simulink library "GenTil_Lib"  (R2023a)
settings: Solver=VariableStepAuto  StartTime=0.0  StopTime=10.0  RelTol=1e-3
values from neighbouring files (symbols this model uses):
  D = [0	0	0	0	0	0	0	0	0	0	0 ... (first row only)    [GenTil.m]
undefined symbols (not defined in the file or in its folder): aircraft, p, phi, psi, q, r, theta, v, w, x, y, z
libraries: simulink_extras x35, simulink x5, matrix_library x4, aerolibatmos2 x1
(part 1 of 2)
settings Model: Creator=igmso  LastModifiedBy=igmso

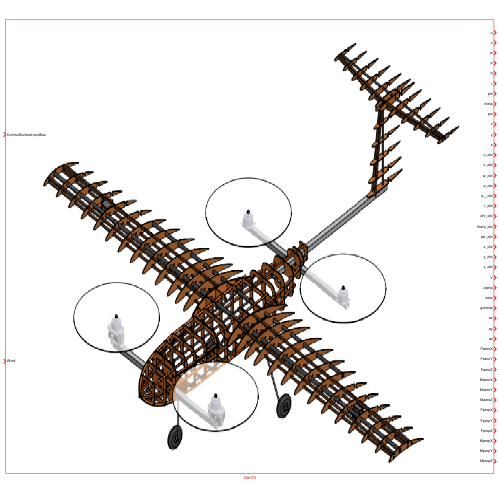
[thumbnail: Simulink's stored preview of the top-level diagram]
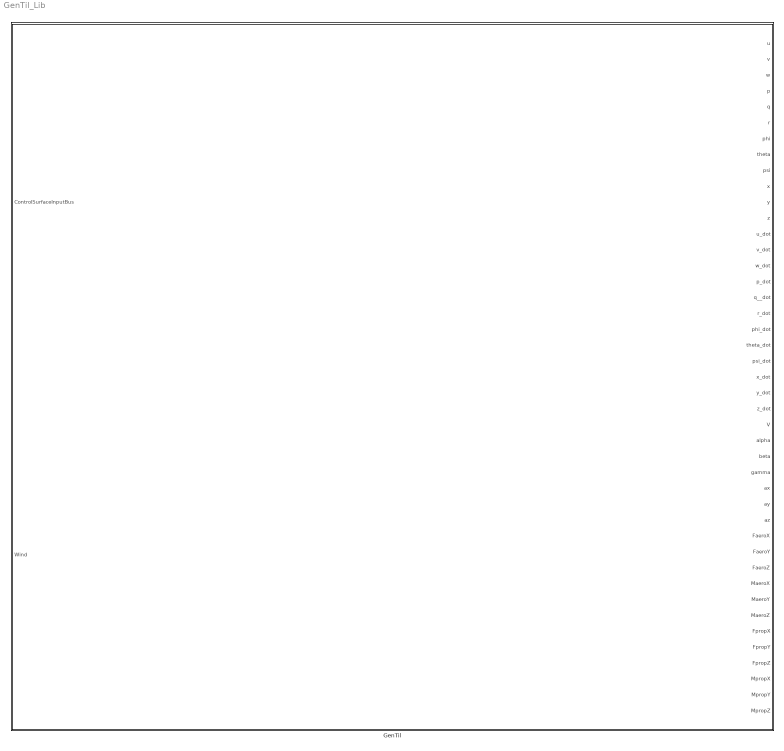
== system GenTil_Lib ==
  GenTil : Subsystem
      mask Display: image('Tilt.png'); % Use "Edit Image" on toolstrip to change.

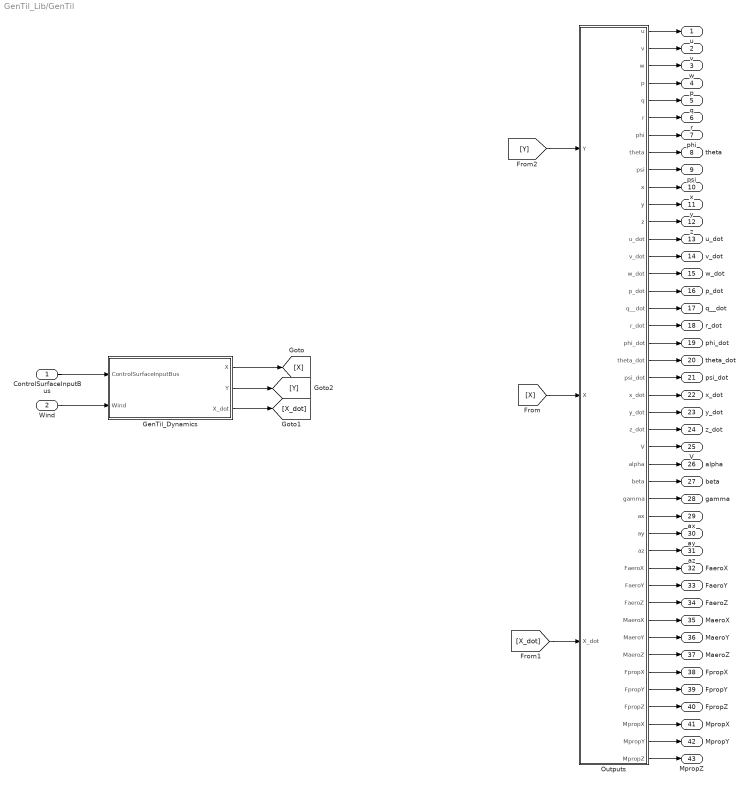
== system GenTil_Lib/GenTil ==
  ControlSurfaceInputBus : Inport  OutDataTypeStr=Bus: Actuators
  Wind : Inport  Port=2
  GenTil_Dynamics : Subsystem
  Outputs : Subsystem
  u : Outport
  v : Outport  Port=2
  w : Outport  Port=3
  p : Outport  Port=4
  q : Outport  Port=5
  r : Outport  Port=6
  phi : Outport  Port=7
  theta : Outport  Port=8
  psi : Outport  Port=9
  x : Outport  Port=10
  y : Outport  Port=11
  z : Outport  Port=12
  u_dot : Outport  Port=13
  v_dot : Outport  Port=14
  w_dot : Outport  Port=15
  p_dot : Outport  Port=16
  q__dot : Outport  Port=17
  r_dot : Outport  Port=18
  phi_dot : Outport  Port=19
  theta_dot : Outport  Port=20
  psi_dot : Outport  Port=21
  x_dot : Outport  Port=22
  y_dot : Outport  Port=23
  z_dot : Outport  Port=24
  V : Outport  Port=25
  alpha : Outport  Port=26
  beta : Outport  Port=27
  gamma : Outport  Port=28
  ax : Outport  Port=29
  ay : Outport  Port=30
  az : Outport  Port=31
  FaeroX : Outport  Port=32
  FaeroY : Outport  Port=33
  FaeroZ : Outport  Port=34
  MaeroX : Outport  Port=35
  MaeroY : Outport  Port=36
  MaeroZ : Outport  Port=37
  FpropX : Outport  Port=38
  FpropY : Outport  Port=39
  FpropZ : Outport  Port=40
  MpropX : Outport  Port=41
  MpropY : Outport  Port=42
  MpropZ : Outport  Port=43
  wires:
  Outputs/40(FpropZ) -> FpropZ/1
  Outputs/12(z) -> z/1
  Outputs/8(theta) -> theta/1
  GenTil_Dynamics/1(X) -> [X]
  Outputs/1(u) -> u/1
  Outputs/19(phi_dot) -> phi_dot/1
  Outputs/20(theta_dot) -> theta_dot/1
  Outputs/3(w) -> w/1
  Outputs/27(beta) -> beta/1
  Outputs/39(FpropY) -> FpropY/1
  GenTil_Dynamics/2(Y) -> [Y]
  Outputs/6(r) -> r/1
  Outputs/31(az) -> az/1
  Outputs/33(FaeroY) -> FaeroY/1
  Outputs/23(y_dot) -> y_dot/1
  [X_dot] -> Outputs/3(X_dot)
  Outputs/2(v) -> v/1
  Outputs/9(psi) -> psi/1
  Outputs/30(ay) -> ay/1
  Outputs/41(MpropX) -> MpropX/1
  Outputs/11(y) -> y/1
  Outputs/18(r_dot) -> r_dot/1
  Outputs/34(FaeroZ) -> FaeroZ/1
  Outputs/16(p_dot) -> p_dot/1
  Outputs/24(z_dot) -> z_dot/1
  [Y] -> Outputs/1(Y)
  Outputs/37(MaeroZ) -> MaeroZ/1
  Outputs/43(MpropZ) -> MpropZ/1
  Outputs/35(MaeroX) -> MaeroX/1
  Outputs/13(u_dot) -> u_dot/1
  Outputs/28(gamma) -> gamma/1
  Outputs/26(alpha) -> alpha/1
  Outputs/5(q) -> q/1
  Outputs/42(MpropY) -> MpropY/1
  Outputs/29(ax) -> ax/1
  Outputs/7(phi) -> phi/1
  GenTil_Dynamics/3(X_dot) -> [X_dot]
  [X] -> Outputs/2(X)
  Outputs/22(x_dot) -> x_dot/1
  Outputs/10(x) -> x/1
  Outputs/36(MaeroY) -> MaeroY/1
  Outputs/25(V) -> V/1
  Outputs/4(p) -> p/1
  Outputs/15(w_dot) -> w_dot/1
  Outputs/32(FaeroX) -> FaeroX/1
  ControlSurfaceInputBus/1 -> GenTil_Dynamics/1(ControlSurfaceInputBus)
  Outputs/38(FpropX) -> FpropX/1
  Wind/1 -> GenTil_Dynamics/2(Wind)
  Outputs/21(psi_dot) -> psi_dot/1
  Outputs/17(q__dot) -> q__dot/1
  Outputs/14(v_dot) -> v_dot/1

== system GenTil_Lib/GenTil/GenTil_Dynamics ==
  ControlSurfaceInputBus : Inport  OutDataTypeStr=Bus: Actuators
  Wind : Inport  Port=2
  Add1 : Sum  Inputs=+-
  Bus Creator : BusCreator  Inputs=2
  Bus Creator2 : BusCreator  Inputs=6
  Bus Creator5 : BusCreator  Inputs=19  OutDataTypeStr=Bus: Outs
      settings: InheritFromInputs=off
  Bus Selector : BusSelector  OutputSignals=theta
  Constant : Constant  Value=aircraft.m  OutDataTypeStr=double  SampleTime=-1
  Constant1 : Constant  Value=aircraft.J_O_b  VectorParams1D=off  OutDataTypeStr=double  SampleTime=-1
  Demux{1..2,4..6} (5 alike) : Demux  Outputs=3
  Demux3 : Demux  Outputs=6
  Equations_of_Motion_6DoF : Subsystem
  GenTilAeroProp : Subsystem
  Subsystem : Subsystem
  X : Outport  OutDataTypeStr=Bus: States
  Y : Outport  Port=2  OutDataTypeStr=Bus: Outs
  X_dot : Outport  Port=3
  wires:
  Bus Selector/1 -> [theta]  "<theta>"
  GenTilAeroProp/2(Moments) -> Demux1/1
  Demux6/3 -> Bus Creator2/3  "Zaero"
  Demux6/2 -> Bus Creator2/2  "Yaero"
  Demux1/1 -> Bus Creator2/4  "Laero"
  Constant/1 -> Bus Creator/1  "Mass_kg"
  Demux1/3 -> Bus Creator2/6  "Naero"
  Bus Creator2/1 -> Equations_of_Motion_6DoF/2(FromAero)  "FromAero"
  GenTilAeroProp/3(alpha) -> [alpha]  "alpha"
  GenTilAeroProp/5(V) -> [V]  "V"
  Constant1/1 -> Bus Creator/2  "InertiaTensor"
  ControlSurfaceInputBus/1 -> GenTilAeroProp/2(ControlSurfaceInputBus)  "Actuators"
  Bus Creator/1 -> Equations_of_Motion_6DoF/3(FromGeometry)  "FromGeometry"
  Demux6/1 -> Bus Creator2/1  "Xaero"
  Equations_of_Motion_6DoF/1(X) -> [X], Bus Selector/1  "X"
  GenTilAeroProp/4(beta) -> [beta]  "beta_"
  Wind/1 -> GenTilAeroProp/3(Wind)
  Subsystem/1(FromLG) -> Equations_of_Motion_6DoF/1(FromLG)
  GenTilAeroProp/6(n_C_b) -> [n_C_b]
  Demux5/3 -> Bus Creator5/18  "MpropZ"
  Demux2/1 -> Bus Creator5/4  "ax"
  Demux3/2 -> Bus Creator5/8  "FaeroY"
  Demux3/1 -> Bus Creator5/7  "FaeroX"
  [n_C_b] -> Demux2/1
  Add1/1 -> Bus Creator5/19  "gamma"
  Demux5/2 -> Bus Creator5/17  "MpropY"
  [alpha] -> Bus Creator5/2  "alpha"
  [V] -> Bus Creator5/1  "V"
  [FandM] -> Demux3/1
  Demux3/4 -> Bus Creator5/10  "MaeroX"
  Demux2/3 -> Bus Creator5/6  "az"
  [Fprop] -> Demux4/1
  Demux2/2 -> Bus Creator5/5  "ay"
  Demux5/1 -> Bus Creator5/16  "MpropX"
  Demux4/3 -> Bus Creator5/15  "FpropZ"
  [alpha] -> Add1/2  "alpha"
  [Mprop] -> Demux5/1
  Demux3/6 -> Bus Creator5/12  "MaeroZ"
  Bus Creator5/1 -> Y/1  "Outs"
  [beta] -> Bus Creator5/3  "beta"
  [theta] -> Add1/1
  Demux4/2 -> Bus Creator5/14  "FpropY"
  Demux4/1 -> Bus Creator5/13  "FpropX"
  Demux3/3 -> Bus Creator5/9  "FaeroZ"
  Demux3/5 -> Bus Creator5/11  "MaeroY"
  Equations_of_Motion_6DoF/2(X_dot) -> [Xdot]
  GenTilAeroProp/1(Forces) -> Demux6/1
  GenTilAeroProp/8(Fprop) -> [Fprop]
  GenTilAeroProp/7(Mprop) -> [Mprop]
  GenTilAeroProp/9(AeroCoeficients) -> [FandM]
  Demux1/2 -> Bus Creator2/5  "Maero"
  [X] -> Subsystem/1(X)
  [X] -> GenTilAeroProp/1(X)
  [X] -> X/1
  [Xdot] -> X_dot/1

== system GenTil_Lib/GenTil/Outputs ==
  Y : Inport  OutDataTypeStr=Bus: Outs
  X : Inport  Port=2  OutDataTypeStr=Bus: States
  X_dot : Inport  Port=3
  Bus Selector : BusSelector  OutputSignals=u,v,w,p,q,r,phi,theta,psi,x,y,z
  Bus Selector1 : BusSelector  OutputSignals=V,alpha,beta,gamma,ax,ay,az,FaeroX,FaeroY,FaeroZ,MaeroX,MaeroY,MaeroZ,FpropX,FpropY,FpropZ,MpropX,MpropY,MpropZ
  Demux1 : Demux  Outputs=12
  u : Outport
  v : Outport  Port=2
  w : Outport  Port=3
  p : Outport  Port=4
  q : Outport  Port=5
  r : Outport  Port=6
  phi : Outport  Port=7
  theta : Outport  Port=8
  psi : Outport  Port=9
  x : Outport  Port=10
  y : Outport  Port=11
  z : Outport  Port=12
  u_dot : Outport  Port=13
  v_dot : Outport  Port=14
  w_dot : Outport  Port=15
  p_dot : Outport  Port=16
  q__dot : Outport  Port=17
  r_dot : Outport  Port=18
  phi_dot : Outport  Port=19
  theta_dot : Outport  Port=20
  psi_dot : Outport  Port=21
  x_dot : Outport  Port=22
  y_dot : Outport  Port=23
  z_dot : Outport  Port=24
  V : Outport  Port=25
  alpha : Outport  Port=26
  beta : Outport  Port=27
  gamma : Outport  Port=28
  ax : Outport  Port=29
  ay : Outport  Port=30
  az : Outport  Port=31
  FaeroX : Outport  Port=32
  FaeroY : Outport  Port=33
  FaeroZ : Outport  Port=34
  MaeroX : Outport  Port=35
  MaeroY : Outport  Port=36
  MaeroZ : Outport  Port=37
  FpropX : Outport  Port=38
  FpropY : Outport  Port=39
  FpropZ : Outport  Port=40
  MpropX : Outport  Port=41
  MpropY : Outport  Port=42
  MpropZ : Outport  Port=43
  wires:
  Bus Selector1/4 -> gamma/1  "<gamma>"
  Demux1/8 -> theta_dot/1  "theta_deg_dot"
  Demux1/1 -> u_dot/1  "u_dot"
  Demux1/9 -> psi_dot/1  "psi_deg_dot"
  Demux1/5 -> q__dot/1  "q_deg_s_dot"
  Demux1/12 -> z_dot/1  "z_dot"
  Demux1/7 -> phi_dot/1  "phi_deg_dot"
  Bus Selector/1 -> u/1  "<u>"
  Bus Selector/2 -> v/1  "<v>"
  Bus Selector1/3 -> beta/1  "<beta>"
  Bus Selector1/6 -> ay/1  "<ay>"
  Bus Selector1/8 -> FaeroX/1  "<FaeroX>"
  Demux1/4 -> p_dot/1  "p_deg_s_dot"
  Bus Selector/5 -> q/1  "<q>"
  Demux1/11 -> y_dot/1  "y_dot"
  Bus Selector1/1 -> V/1  "<V>"
  Bus Selector/12 -> z/1  "<z>"
  Bus Selector1/12 -> MaeroY/1  "<MaeroY>"
  Bus Selector/11 -> y/1  "<y>"
  Bus Selector/6 -> r/1  "<r>"
  Y/1 -> Bus Selector1/1
  Bus Selector1/15 -> FpropY/1  "<FpropY>"
  Bus Selector1/10 -> FaeroZ/1  "<FaeroZ>"
  X_dot/1 -> Demux1/1
  Bus Selector/8 -> theta/1  "<theta>"
  Bus Selector1/9 -> FaeroY/1  "<FaeroY>"
  Bus Selector1/2 -> alpha/1  "<alpha>"
  Bus Selector1/5 -> ax/1  "<ax>"
  Bus Selector/4 -> p/1  "<p>"
  Demux1/2 -> v_dot/1  "v_dot"
  Bus Selector1/19 -> MpropZ/1  "<MpropZ>"
  Demux1/10 -> x_dot/1  "x_dot"
  Demux1/3 -> w_dot/1  "w_dot"
  Bus Selector/7 -> phi/1  "<phi>"
  Bus Selector/9 -> psi/1  "<psi>"
  Demux1/6 -> r_dot/1  "r_deg_s_dot"
  Bus Selector1/17 -> MpropX/1  "<MpropX>"
  Bus Selector1/16 -> FpropZ/1  "<FpropZ>"
  Bus Selector1/18 -> MpropY/1  "<MpropY>"
  X/1 -> Bus Selector/1
  Bus Selector/10 -> x/1  "<x>"
  Bus Selector1/14 -> FpropX/1  "<FpropX>"
  Bus Selector/3 -> w/1  "<w>"
  Bus Selector1/7 -> az/1  "<az>"
  Bus Selector1/13 -> MaeroZ/1  "<MaeroZ>"
  Bus Selector1/11 -> MaeroX/1  "<MaeroX>"

== system GenTil_Lib/GenTil/GenTil_Dynamics/Equations_of_Motion_6DoF ==
  FromLG : Inport
  FromAero : Inport  Port=2
  FromGeometry : Inport  Port=3
  " " : Subsystem
  Bus Creator1 : BusCreator  Inputs=u,v,w,p,q,r,phi,theta,psi,x,y,z  OutDataTypeStr=Bus: States
  Bus Selector : BusSelector  OutputSignals=Fz_LG_N
  Bus Selector1 : BusSelector  OutputSignals=Xaero,Yaero,Zaero,Laero,Maero,Naero
  Demux : Demux  Outputs=2
  Demux1 : Demux  Outputs=12
  Dynamics : Subsystem
  Min : MinMax  Inputs=2
  Mux1 : Mux  Inputs=6
  p : Integrator  InitialCondition=aircraft.Trim.p  ContinuousStateAttributes='p'
  phi : Integrator  InitialCondition=aircraft.Trim.phi  ContinuousStateAttributes='phi'
  psi : Integrator  InitialCondition=aircraft.Trim.psi  ContinuousStateAttributes='psi'
  q : Integrator  InitialCondition=aircraft.Trim.q  ContinuousStateAttributes='q'
  r : Integrator  InitialCondition=aircraft.Trim.r  ContinuousStateAttributes='r'
  theta : Integrator  InitialCondition=aircraft.Trim.theta  ContinuousStateAttributes='theta'
  u : Integrator  InitialCondition=aircraft.Trim.u  ContinuousStateAttributes='u'
  v : Integrator  InitialCondition=aircraft.Trim.v  ContinuousStateAttributes='v'
  w : Integrator  InitialCondition=aircraft.Trim.w  ContinuousStateAttributes='w'
  x : Integrator  InitialCondition=aircraft.Trim.x  ContinuousStateAttributes='x'
  y : Integrator  InitialCondition=aircraft.Trim.y  ContinuousStateAttributes='y'
  z : Integrator  InitialCondition=aircraft.Trim.z  ContinuousStateAttributes='z'
  X : Outport  OutDataTypeStr=Bus: States
  X_dot : Outport  Port=2
  wires:
  [ZG] -> Min/1
  Bus Selector/1 -> [ZG]  "<Fz_LG_N>"
  [MA] -> " "/2(MA)
  [z] -> " "/1(z)
  [ZA] -> Min/2
  [YA] -> Mux1/2
  [XA] -> Mux1/1
  [NA] -> Mux1/6
  [LA] -> Mux1/4
  " "/1(Out) -> Mux1/5
  Bus Selector1/6 -> [NA]  "<Naero>"
  Bus Selector1/5 -> [MA]  "<Maero>"
  Bus Selector1/4 -> [LA]  "<Laero>"
  Bus Selector1/3 -> [ZA]  "<Zaero>"
  Bus Selector1/2 -> [YA]  "<Yaero>"
  Bus Selector1/1 -> [XA]  "<Xaero>"
  Demux/2 -> Dynamics/4(Moments_Nm)  "Moments_Nm"
  Demux/1 -> Dynamics/3(Forces_N)  "Forces_N"
  Min/1 -> Mux1/3
  Mux1/1 -> Demux/1
  FromAero/1 -> Bus Selector1/1
  FromLG/1 -> Bus Selector/1
  Dynamics/1(X_dot) -> [Xdot], Demux1/1  "X_dot"
  Demux1/12 -> z/1  "z_dot"
  Demux1/4 -> p/1  "p_deg_s_dot"
  Demux1/10 -> x/1  "x_dot"
  theta/1 -> Bus Creator1/8  "theta"
  Demux1/9 -> psi/1  "psi_deg_dot"
  Demux1/2 -> v/1  "v_dot"
  Demux1/3 -> w/1  "w_dot"
  Demux1/11 -> y/1  "y_dot"
  Demux1/8 -> theta/1  "theta_deg_dot"
  Demux1/1 -> u/1  "u_dot"
  Demux1/5 -> q/1  "q_deg_s_dot"
  psi/1 -> Bus Creator1/9  "psi"
  w/1 -> Bus Creator1/3  "w"
  phi/1 -> Bus Creator1/7  "phi"
  q/1 -> Bus Creator1/5  "q"
  Bus Creator1/1 -> [X], X/1  "X"
  v/1 -> Bus Creator1/2  "v"
  z/1 -> [z], Bus Creator1/12  "z"
  p/1 -> Bus Creator1/4  "p"
  Demux1/6 -> r/1  "r_deg_s_dot"
  u/1 -> Bus Creator1/1  "u"
  r/1 -> Bus Creator1/6  "r"
  Demux1/7 -> phi/1  "phi_deg_dot"
  x/1 -> Bus Creator1/10  "x"
  y/1 -> Bus Creator1/11  "y"
  FromGeometry/1 -> [mass]
  [X] -> Dynamics/2(X)
  [mass] -> Dynamics/1(FromGeometry)
  [Xdot] -> X_dot/1

== system GenTil_Lib/GenTil/GenTil_Dynamics/GenTilAeroProp ==
  X : Inport  OutDataTypeStr=Bus: States
  ControlSurfaceInputBus : Inport  Port=2  OutDataTypeStr=Bus: Actuators
  Wind : Inport  Port=3
  Add : Sum
  Add1 : Sum
  Aerodynamics : Subsystem
  Bus Selector : BusSelector  OutputSignals=z
  Constant1 : Constant  SampleTime=-1
  Constant2 : Constant  Value=aircraft.m  SampleTime=-1
  Divide : Product  Inputs=*/
  Gain : Gain  Gain=-1
  ISA Atmosphere Model : aerolibatmos2/ISA Atmosphere Model  custom=off  g=9.80665  gamma=1.4  R=287.0531  L=0.0065  h_trop=11000  h_strat=20000  rho0=1.225  P0=101325  T0=288.15  h0=0
  Product : Product
  PropLoads : Subsystem
  Terminator : Terminator
  Terminator1 : Terminator
  Terminator2 : Terminator
  Forces : Outport
  Moments : Outport  Port=2
  alpha : Outport  Port=3
  beta : Outport  Port=4
  V : Outport  Port=5
  n_C_b : Outport  Port=6
  Mprop : Outport  Port=7
  Fprop : Outport  Port=8
  AeroCoeficients : Outport  Port=9
  wires:
  ISA Atmosphere Model/1 -> Terminator1/1
  ISA Atmosphere Model/2 -> Terminator/1
  Add/1 -> Forces/1, [Forces]  "Forces"
  Add1/1 -> Moments/1  "Moments"
  PropLoads/2(Fprop) -> [Fprop]
  ISA Atmosphere Model/3 -> Terminator2/1
  Bus Selector/1 -> Gain/1  "<z>"
  Gain/1 -> ISA Atmosphere Model/1
  Aerodynamics/2(Faero) -> [Faero]
  [Wind] -> Aerodynamics/3(Wind)
  Divide/1 -> Product/1
  Product/1 -> n_C_b/1
  [Forces] -> Product/2
  Constant1/1 -> Divide/1
  Constant2/1 -> Divide/2
  Wind/1 -> [Wind]
  X/1 -> [X]
  ControlSurfaceInputBus/1 -> [ControlSurface]
  [X] -> Bus Selector/1
  ISA Atmosphere Model/4 -> Aerodynamics/2(AirDensity)
  [ControlSurface] -> Aerodynamics/1(ControlSurfaceInputBus), PropLoads/1(ControlInputBus)
  [X] -> Aerodynamics/4(X)
  PropLoads/1(Mprop_O_b) -> [MProp]
  Aerodynamics/3(alpha_deg) -> alpha/1
  Aerodynamics/4(beta_deg) -> beta/1
  Aerodynamics/1(Maero) -> [Maero]
  Aerodynamics/6(AeroCoeficients) -> [FandM]
  Aerodynamics/5(V) -> V/1
  [Faero] -> Add/1
  [Fprop] -> Add/2
  [Maero] -> Add1/1
  [MProp] -> Add1/2
  [MProp] -> Mprop/1
  [Fprop] -> Fprop/1
  [FandM] -> AeroCoeficients/1

== system GenTil_Lib/GenTil/GenTil_Dynamics/Subsystem ==
  X : Inport
  Bus Creator1 : BusCreator  Inputs=6
  Bus Selector3 : BusSelector  OutputSignals=z
  Compare To Constant : simulink/Logic and Bit Operations/Compare To Constant  relop=>=  const=-0.05  OutDataTypeStr=boolean
  Constant1 : Constant  Value=-aircraft.g*aircraft.m
  Constant{2..3,5..7} (5 alike) : Constant  Value=0
  Data Type Conversion : DataTypeConversion  OutDataTypeStr=double  SaturateOnIntegerOverflow=off  RndMeth=Floor
  Product : Product
  FromLG : Outport
  wires:
  Constant5/1 -> Bus Creator1/4  "Mx_LG_Nm"
  Constant2/1 -> Bus Creator1/1  "Fx_LG_N"
  Bus Creator1/1 -> FromLG/1  "FromLG"
  Constant6/1 -> Bus Creator1/5  "My_LG_Nm"
  Constant7/1 -> Bus Creator1/6  "Mz_LG_Nm"
  Constant3/1 -> Bus Creator1/2  "Fy_LG_N"
  Product/1 -> Bus Creator1/3  "Fz_LG_N"
  Bus Selector3/1 -> Compare To Constant/1  "<z>"
  Constant1/1 -> Product/1
  Compare To Constant/1 -> Data Type Conversion/1
  Data Type Conversion/1 -> Product/2
  X/1 -> Bus Selector3/1

== system GenTil_Lib/GenTil/GenTil_Dynamics/Equations_of_Motion_6DoF/  ==
  z : Inport
  MA : Inport  Port=2
  Compare To Constant : simulink/Logic and Bit Operations/Compare To Constant  relop=<=  const=-0.05  OutDataTypeStr=boolean
  Constant : Constant  Value=0  SampleTime=-1
  Data Type Conversion : DataTypeConversion  OutDataTypeStr=double  SaturateOnIntegerOverflow=off  RndMeth=Floor
  Switch : Switch  Criteria=u2 > Threshold  Threshold=0.05  SaturateOnIntegerOverflow=off  InputSameDT=off
  Out : Outport
  wires:
  Constant/1 -> Switch/3
  Switch/1 -> Out/1
  Compare To Constant/1 -> Data Type Conversion/1
  MA/1 -> Switch/1
  Data Type Conversion/1 -> Switch/2
  z/1 -> Compare To Constant/1

== system GenTil_Lib/GenTil/GenTil_Dynamics/Equations_of_Motion_6DoF/Dynamics ==
  FromGeometry : Inport  OutDataTypeStr=double
  X : Inport  Port=2  OutDataTypeStr=Bus: States  PortDimensions=12
  Forces_N : Inport  Port=3  OutDataTypeStr=double  PortDimensions=[3,1]
  Moments_Nm : Inport  Port=4  OutDataTypeStr=double  PortDimensions=[3,1]
  Accelerations : Subsystem
  Bus Creator2 : BusCreator  Inputs=3
  Bus Selector1 : BusSelector  OutputSignals=phi,theta,psi
  Degrees to Radians3 : simulink_extras/Transformations/Degrees to Radians
  Degrees to Radians4 : simulink_extras/Transformations/Degrees to Radians
  Degrees to Radians5 : simulink_extras/Transformations/Degrees to Radians
  Forces : Subsystem
  Generalized Mass Matrix : Subsystem
  Matrix Concatenate : Concatenate  Mode=Multidimensional array
  Moments : Subsystem
  Mux : Mux  Inputs=3
  Rotation Matrix : Subsystem
  Translational and Rotational Kinematics : Subsystem
  X_dot : Outport
  wires:
  [M_b] -> Matrix Concatenate/2
  [F_b] -> Matrix Concatenate/1
  Rotation Matrix/2(C_phi) -> Translational and Rotational Kinematics/3(C_phi)
  Rotation Matrix/1(C_bv) -> Translational and Rotational Kinematics/2(C_bv)  "C_bv"
  Bus Selector1/2 -> Degrees to Radians4/1  "<theta>"
  Translational and Rotational Kinematics/2(dReodt) -> Mux/3  "dReodt"
  Generalized Mass Matrix/1(Mgen) -> [Mgen]  "Mgen"
  Degrees to Radians4/1 -> Bus Creator2/2  "theta_rad"
  Accelerations/1(e_dot) -> Mux/1  "e_dot"
  Bus Selector1/1 -> Degrees to Radians3/1  "<phi>"
  Bus Selector1/3 -> Degrees to Radians5/1  "<psi>"
  Degrees to Radians5/1 -> Bus Creator2/3  "psi_rad"
  Translational and Rotational Kinematics/1(Phi_dot) -> Mux/2  "Phi_dot"
  Degrees to Radians3/1 -> Bus Creator2/1  "phi_rad"
  Matrix Concatenate/1 -> Accelerations/2(F_and_M)  "[F_b;M_b]"
  Bus Creator2/1 -> [att_rad]
  Mux/1 -> X_dot/1  "X_dot"
  Forces/1(F_b) -> [F_b]
  Moments/1(M_b) -> [M_b]
  X/1 -> [X]
  FromGeometry/1 -> [mass]
  Forces_N/1 -> [F]
  Moments_Nm/1 -> [M]
  [X] -> Bus Selector1/1
  [X] -> Translational and Rotational Kinematics/1(X)
  [X] -> Forces/1(X)
  [F] -> Forces/2(Forces_N)
  [mass] -> Moments/1(FromGeometry), Generalized Mass Matrix/1(FromGeometry), Forces/3(FromGeometry)
  [X] -> Moments/2(X)
  [M] -> Moments/3(Moments_Nm)
  [Mgen] -> Accelerations/1(Mgen)
  [att_rad] -> Rotation Matrix/1(attitude_angles_rad)

== system GenTil_Lib/GenTil/GenTil_Dynamics/GenTilAeroProp/Aerodynamics ==
  ControlSurfaceInputBus : Inport  OutDataTypeStr=Bus: Actuators
  AirDensity : Inport  Port=2
  Wind : Inport  Port=3
  X : Inport  Port=4  OutDataTypeStr=Bus: States
  Aero_Loads_GTVTOL : Subsystem
  Aerodynamic_System : Subsystem
  Maero : Outport
  Faero : Outport  Port=2
  alpha_deg : Outport  Port=3
  beta_deg : Outport  Port=4
  V : Outport  Port=5
  AeroCoeficients : Outport  Port=6
  wires:
  ControlSurfaceInputBus/1 -> Aero_Loads_GTVTOL/7(ControlSurfaceInputBus)
  AirDensity/1 -> Aero_Loads_GTVTOL/1(AirDensity)
  Aerodynamic_System/4(C_ba) -> Aero_Loads_GTVTOL/6(C_ba)
  X/1 -> Aero_Loads_GTVTOL/2(X), Aerodynamic_System/1(X)
  Aero_Loads_GTVTOL/1(Faero) -> Faero/1
  Aero_Loads_GTVTOL/2(Maero) -> Maero/1
  Wind/1 -> Aerodynamic_System/2(Wind)
  Aero_Loads_GTVTOL/3(AeroCoeficients) -> AeroCoeficients/1
  Aerodynamic_System/5(V) -> [V]
  Aerodynamic_System/1(V_rel) -> Aero_Loads_GTVTOL/3(V_rel)
  Aerodynamic_System/2(alpha_deg) -> [alpha], Aero_Loads_GTVTOL/4(alpha_deg)
  Aerodynamic_System/3(beta_deg) -> [beta], Aero_Loads_GTVTOL/5(beta_deg)
  [V] -> V/1
  [alpha] -> alpha_deg/1
  [beta] -> beta_deg/1

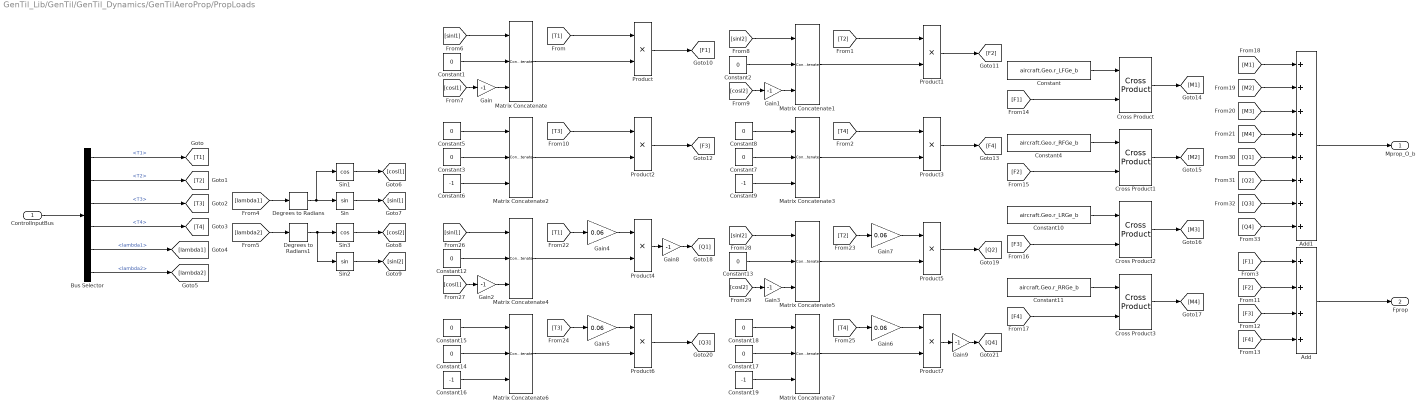
== system GenTil_Lib/GenTil/GenTil_Dynamics/GenTilAeroProp/PropLoads ==
  ControlInputBus : Inport  OutDataTypeStr=Bus: Actuators
  Add : Sum  Inputs=++++
  Add1 : Sum  Inputs=8
  Bus Selector : BusSelector  OutputSignals=T1,T2,T3,T4,lambda1,lambda2
  Constant : Constant  Value=aircraft.Geo.r_LFGe_b  SampleTime=-1
  Constant{1..3,5,7..8,12..15,17..18} (12 alike) : Constant  Value=0  SampleTime=-1
  Constant10 : Constant  Value=aircraft.Geo.r_LRGe_b  SampleTime=-1
  Constant11 : Constant  Value=aircraft.Geo.r_RRGe_b  SampleTime=-1
  Constant{6,9,16,19} (4 alike) : Constant  Value=-1  SampleTime=-1
  Constant4 : Constant  Value=aircraft.Geo.r_RFGe_b  SampleTime=-1
  Cross Product{,1..3} (4 alike) : matrix_library/Cross Product
  Degrees to Radians : simulink_extras/Transformations/Degrees to Radians
  Degrees to Radians1 : simulink_extras/Transformations/Degrees to Radians
  Gain{,1..3,8..9} (6 alike) : Gain  Gain=-1
  Gain{4..7} (4 alike) : Gain  Gain=0.06
  Matrix Concatenate{,1..7} (8 alike) : Concatenate  NumInputs=3  Mode=Multidimensional array
  Product{,1..7} (8 alike) : Product
  Sin : Trigonometry
  Sin1 : Trigonometry  Operator=cos
  Sin2 : Trigonometry
  Sin3 : Trigonometry  Operator=cos
  Mprop_O_b : Outport
  Fprop : Outport  Port=2
  wires:
  Bus Selector/5 -> [lambda1]  "<lambda1>"
  Add1/1 -> Mprop_O_b/1
  Bus Selector/3 -> [T3]  "<T3>"
  Bus Selector/4 -> [T4]  "<T4>"
  Bus Selector/2 -> [T2]  "<T2>"
  ControlInputBus/1 -> Bus Selector/1
  Bus Selector/1 -> [T1]  "<T1>"
  Add/1 -> Fprop/1
  Bus Selector/6 -> [lambda2]  "<lambda2>"
  [lambda1] -> Degrees to Radians/1
  [lambda2] -> Degrees to Radians1/1
  Degrees to Radians/1 -> Sin1/1, Sin/1
  Sin1/1 -> [cosl1]
  Sin/1 -> [sinl1]
  Sin2/1 -> [sinl2]
  Sin3/1 -> [cosl2]
  Degrees to Radians1/1 -> Sin2/1, Sin3/1
  [sinl1] -> Matrix Concatenate/1
  [cosl1] -> Gain/1
  Gain/1 -> Matrix Concatenate/3
  Constant1/1 -> Matrix Concatenate/2
  Constant2/1 -> Matrix Concatenate1/2
  Gain1/1 -> Matrix Concatenate1/3
  [cosl2] -> Gain1/1
  [sinl2] -> Matrix Concatenate1/1
  Matrix Concatenate/1 -> Product/2
  [T1] -> Product/1
  [T2] -> Product1/1
  Matrix Concatenate1/1 -> Product1/2
  Product/1 -> [F1]
  Product1/1 -> [F2]
  Product3/1 -> [F4]
  Product2/1 -> [F3]
  Matrix Concatenate3/1 -> Product3/2
  [T4] -> Product3/1
  [T3] -> Product2/1
  Matrix Concatenate2/1 -> Product2/2
  Constant3/1 -> Matrix Concatenate2/2
  Constant6/1 -> Matrix Concatenate2/3
  Constant5/1 -> Matrix Concatenate2/1
  Constant8/1 -> Matrix Concatenate3/1
  Constant7/1 -> Matrix Concatenate3/2
  Constant9/1 -> Matrix Concatenate3/3
  [F1] -> Add/1
  [F2] -> Add/2
  [F3] -> Add/3
  [F4] -> Add/4
  Constant/1 -> Cross Product/1
  [F1] -> Cross Product/2
  [F2] -> Cross Product1/2
  Constant4/1 -> Cross Product1/1
  Constant11/1 -> Cross Product3/1
  [F4] -> Cross Product3/2
  [F3] -> Cross Product2/2
  Constant10/1 -> Cross Product2/1
  Cross Product/1 -> [M1]
  Cross Product1/1 -> [M2]
  Cross Product2/1 -> [M3]
  Cross Product3/1 -> [M4]
  [M1] -> Add1/1
  [M2] -> Add1/2
  [M3] -> Add1/3
  [M4] -> Add1/4
  Constant19/1 -> Matrix Concatenate7/3
  Constant17/1 -> Matrix Concatenate7/2
  Constant18/1 -> Matrix Concatenate7/1
  Constant15/1 -> Matrix Concatenate6/1
  Constant16/1 -> Matrix Concatenate6/3
  Constant14/1 -> Matrix Concatenate6/2
  Matrix Concatenate6/1 -> Product6/2
  [T3] -> Gain5/1
  [T4] -> Gain6/1
  Matrix Concatenate7/1 -> Product7/2
  Product6/1 -> [Q3]
  Product5/1 -> [Q2]
  Product4/1 -> Gain8/1
  Matrix Concatenate5/1 -> Product5/2
  [T2] -> Gain7/1
  [T1] -> Gain4/1
  Matrix Concatenate4/1 -> Product4/2
  [sinl2] -> Matrix Concatenate5/1
  [cosl2] -> Gain3/1
  Gain3/1 -> Matrix Concatenate5/3
  Constant13/1 -> Matrix Concatenate5/2
  Constant12/1 -> Matrix Concatenate4/2
  Gain2/1 -> Matrix Concatenate4/3
  [cosl1] -> Gain2/1
  [sinl1] -> Matrix Concatenate4/1
  Gain4/1 -> Product4/1
  Gain5/1 -> Product6/1
  Gain6/1 -> Product7/1
  Gain7/1 -> Product5/1
  [Q1] -> Add1/5
  [Q2] -> Add1/6
  [Q3] -> Add1/7
  [Q4] -> Add1/8
  Gain8/1 -> [Q1]
  Product7/1 -> Gain9/1
  Gain9/1 -> [Q4]

== system GenTil_Lib/GenTil/GenTil_Dynamics/Equations_of_Motion_6DoF/Dynamics/Accelerations ==
  Mgen : Inport
  F_and_M : Inport  Port=2
  Demux1 : Demux  Outputs=6
  Divide : Product  Inputs=*/  Multiplication=Matrix(*)
  IdentityMatrix : IdentityMatrix  OutputDimensions=6
  Matrix Multiply : Product  Multiplication=Matrix(*)
  Mux : Mux  Inputs=6
  Radians to Degrees : simulink_extras/Transformations/Radians to Degrees
  Radians to Degrees1 : simulink_extras/Transformations/Radians to Degrees
  Radians to Degrees2 : simulink_extras/Transformations/Radians to Degrees
  e_dot : Outport
  wires:
  Radians to Degrees1/1 -> Mux/5  "theta_dot"
  Demux1/2 -> Mux/2  "v_dot"
  IdentityMatrix/1 -> Divide/1
  Demux1/1 -> Mux/1  "u_dot"
  Demux1/6 -> Radians to Degrees2/1
  F_and_M/1 -> Matrix Multiply/2
  Demux1/3 -> Mux/3  "z_dot"
  Mgen/1 -> Divide/2
  Radians to Degrees2/1 -> Mux/6  "psi_dot"
  Matrix Multiply/1 -> Demux1/1
  Demux1/5 -> Radians to Degrees1/1
  Radians to Degrees/1 -> Mux/4  "phi_dot"
  Divide/1 -> Matrix Multiply/1
  Demux1/4 -> Radians to Degrees/1
  Mux/1 -> e_dot/1  "e_dot"

== system GenTil_Lib/GenTil/GenTil_Dynamics/Equations_of_Motion_6DoF/Dynamics/Forces ==
  note: (m*skew(omega_b)*V_b - m*skew(omega_b)*skew(rC_b)*omega_b)
  X : Inport  OutDataTypeStr=Bus: States  PortDimensions=12
  Forces_N : Inport  Port=2  OutDataTypeStr=double  PortDimensions=[3,1]
  FromGeometry : Inport  Port=3  OutDataTypeStr=double
  Add : Sum  Inputs=+++
  Avoid_Low_Values : Subsystem
  Bus Creator2 : BusCreator  Inputs=3
  Bus Selector : BusSelector  OutputSignals=p,q,r
  Bus Selector1 : BusSelector  OutputSignals=phi,theta,psi
  Bus Selector2 : BusSelector  OutputSignals=Mass_kg
  Bus Selector3 : BusSelector  OutputSignals=u,v,w
  Center of Mass to Origin [m] : Constant  Value=aircraft.rC_b
  Degrees to Radians{,1..5} (6 alike) : simulink_extras/Transformations/Degrees to Radians
  Gain3 : Gain  Gain=-1
  Minus : Sum  Inputs=+-
  Mux : Mux  Inputs=3
  Mux1 : Mux  Inputs=3
  Product : Product  Multiplication=Matrix(*)
  Product1 : Product
  Product3 : Product  Multiplication=Matrix(*)  OutDataTypeStr=double
  Product4 : Product
  Product5 : Product  Inputs=3  Multiplication=Matrix(*)
  Rotation Matrix : Subsystem
  Skew : Subsystem
  Skew1 : Subsystem
  Transpose : Reshape  OutputDimensionality=Column vector (2-D)
  gravity [m/s^2] : Constant  Value=[0;0;aircraft.g]
  F_b : Outport  OutDataTypeStr=double  PortDimensions=[3,1]
  wires:
  Product3/1 -> Minus/1
  Transpose/1 -> Product3/2  "V_b.'"
  [V_b] -> Transpose/1
  [m_skew_wb] -> Product3/1  "m*skew(omega_b)"
  Center of Mass to Origin [m]/1 -> Skew1/1(X)  "rC_b"
  Product5/1 -> Minus/2
  Skew1/1(skew(x)) -> Product5/2  "skew(rC_b)"
  [omega_b] -> Product5/3  "omega_b"
  [m_skew_wb] -> Product5/1  "m*skew(omega_b)"
  [Mass_kg] -> Product1/2
  Bus Selector2/1 -> [Mass_kg]  "<Mass_kg>"
  FromGeometry/1 -> Bus Selector2/1
  Gain3/1 -> Add/2
  Minus/1 -> Gain3/1
  Rotation Matrix/1(C_bv) -> Product/1  "C_bv"
  Bus Selector1/1 -> Degrees to Radians3/1  "<phi>"
  Bus Selector1/2 -> Degrees to Radians4/1  "<theta>"
  Bus Creator2/1 -> [att_rad]  "attitude_angles_rad"
  gravity [m/s^2]/1 -> Product/2  "g"
  Degrees to Radians3/1 -> Bus Creator2/1  "phi_rad"
  Product/1 -> Product1/1  "g_b"
  Bus Selector1/3 -> Degrees to Radians5/1  "<psi>"
  Degrees to Radians5/1 -> Bus Creator2/3  "psi_rad"
  Degrees to Radians4/1 -> Bus Creator2/2  "theta_rad"
  Degrees to Radians/1 -> Mux/1  "p_rad_s"
  Mux/1 -> [omega_b]  "omega_b"
  Bus Selector3/3 -> Mux1/3  "<w>"
  Bus Selector/3 -> Degrees to Radians2/1  "<r>"
  Bus Selector/1 -> Degrees to Radians/1  "<p>"
  Degrees to Radians1/1 -> Mux/2  "q_rad_s"
  Bus Selector/2 -> Degrees to Radians1/1  "<q>"
  Bus Selector3/2 -> Mux1/2  "<v>"
  Degrees to Radians2/1 -> Mux/3  "r_rad_s"
  Bus Selector3/1 -> Mux1/1  "<u>"
  Mux1/1 -> [V_b]  "V_b"
  Product1/1 -> Add/3  "m*g_b"
  X/1 -> [X]
  Forces_N/1 -> [F]
  [X] -> Bus Selector/1, Bus Selector1/1, Bus Selector3/1
  [omega_b] -> Skew/1(X)
  Skew/1(skew(x)) -> Product4/2  "skew(omega_b)"
  [Mass_kg] -> Product4/1
  Product4/1 -> [m_skew_wb]
  [att_rad] -> Rotation Matrix/1(attitude_angles_rad)
  [F] -> Add/1
  Add/1 -> Avoid_Low_Values/1(In)
  Avoid_Low_Values/1(Out) -> F_b/1

== system GenTil_Lib/GenTil/GenTil_Dynamics/Equations_of_Motion_6DoF/Dynamics/Generalized Mass Matrix ==
  FromGeometry : Inport  OutDataTypeStr=double
  3 : IdentityMatrix  OutputDimensions=3
  Bus Selector2 : BusSelector  OutputSignals=Mass_kg,InertiaTensor
  Center of Mass to Origin [m] : Constant  Value=aircraft.rC_b
  Gain : Gain  Gain=-1
  Matrix Concatenate : Concatenate  Mode=Multidimensional array  ConcatenateDimension=2
  Matrix Concatenate1 : Concatenate  Mode=Multidimensional array  ConcatenateDimension=2
  Matrix Concatenate2 : Concatenate  Mode=Multidimensional array
  Product : Product
  Product1 : Product
  Skew : Subsystem
  Mgen : Outport  OutDataTypeStr=double  PortDimensions=[6,6]
  wires:
  Gain/1 -> Matrix Concatenate/2  "-m*skew(rC_b)"
  [Mass_kg] -> Product/1
  Bus Selector2/2 -> [InertiaTensor]  "<InertiaTensor>"
  FromGeometry/1 -> Bus Selector2/1
  Bus Selector2/1 -> [Mass_kg]  "<Mass_kg>"
  [mskew] -> Gain/1
  [mskew] -> Matrix Concatenate1/1  "m*skew(rC_b)"
  Matrix Concatenate2/1 -> Mgen/1  "Mgen"
  Matrix Concatenate/1 -> Matrix Concatenate2/1  "[m*I3 -m*skew(rC_b)]"
  Product/1 -> Matrix Concatenate/1  "m*I3"
  Matrix Concatenate1/1 -> Matrix Concatenate2/2  "[m*skew(rC_b) J_O_b]"
  3/1 -> Product/2  "I3"
  [InertiaTensor] -> Matrix Concatenate1/2  "J_O_b"
  Center of Mass to Origin [m]/1 -> Skew/1(X)
  Skew/1(skew(x)) -> Product1/2  "skew(rC_b)"
  [Mass_kg] -> Product1/1
  Product1/1 -> [mskew]

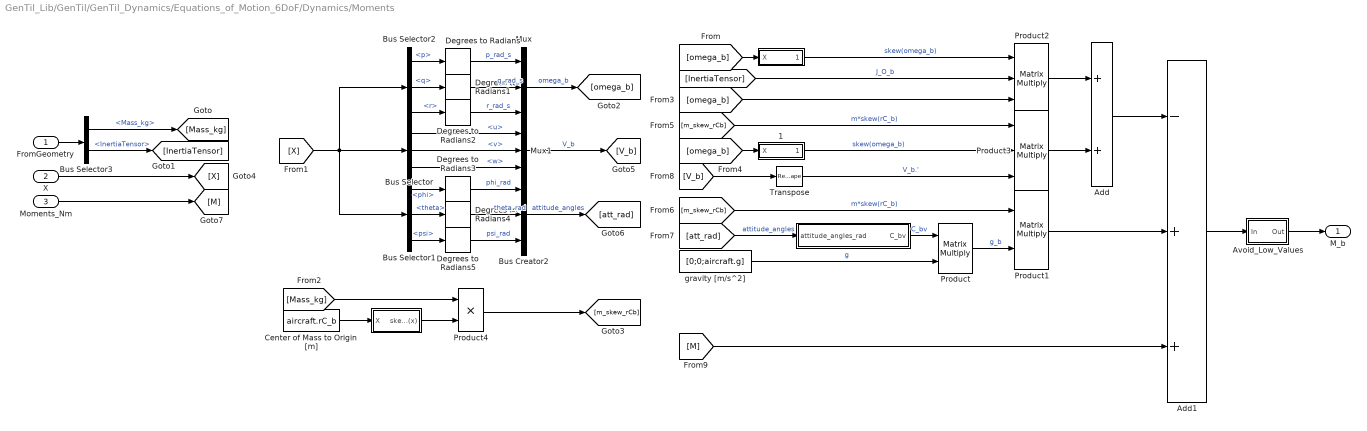
== system GenTil_Lib/GenTil/GenTil_Dynamics/Equations_of_Motion_6DoF/Dynamics/Moments ==
  FromGeometry : Inport  OutDataTypeStr=double
  X : Inport  Port=2  OutDataTypeStr=Bus: States  PortDimensions=12
  Moments_Nm : Inport  Port=3  OutDataTypeStr=double  PortDimensions=[3;1]
  " " : Subsystem
  "  " : Subsystem
  "     " : Subsystem
  " 1" : Subsystem
  Add : Sum
  Add1 : Sum  Inputs=-++
  Avoid_Low_Values : Subsystem
  Bus Creator2 : BusCreator  Inputs=3
  Bus Selector : BusSelector  OutputSignals=u,v,w
  Bus Selector1 : BusSelector  OutputSignals=phi,theta,psi
  Bus Selector2 : BusSelector  OutputSignals=p,q,r
  Bus Selector3 : BusSelector  OutputSignals=Mass_kg,InertiaTensor
  Center of Mass to Origin [m] : Constant  Value=aircraft.rC_b
  Degrees to Radians{,1..5} (6 alike) : simulink_extras/Transformations/Degrees to Radians
  Mux : Mux  Inputs=3
  Mux1 : Mux  Inputs=3
  Product : Product  Multiplication=Matrix(*)
  Product1 : Product  Multiplication=Matrix(*)
  Product2 : Product  Inputs=3  Multiplication=Matrix(*)
  Product3 : Product  Inputs=3  Multiplication=Matrix(*)  OutDataTypeStr=double
  Product4 : Product
  Transpose : Reshape  OutputDimensionality=Column vector (2-D)
  gravity [m/s^2] : Constant  Value=[0;0;aircraft.g]
  M_b : Outport  OutDataTypeStr=double  PortDimensions=[3;1]
  wires:
  Bus Selector3/2 -> [InertiaTensor]  "<InertiaTensor>"
  FromGeometry/1 -> Bus Selector3/1
  Bus Selector3/1 -> [Mass_kg]  "<Mass_kg>"
  [m_skew_rCb] -> Product3/1  "m*skew(rC_b)"
  Degrees to Radians/1 -> Mux/1  "p_rad_s"
  Product1/1 -> Add1/2
  [att_rad] -> "     "/1(attitude_angles_rad)  "attitude_angles"
  Bus Selector1/1 -> Degrees to Radians3/1  "<phi>"
  Bus Selector1/3 -> Degrees to Radians5/1  "<psi>"
  Degrees to Radians5/1 -> Bus Creator2/3  "psi_rad"
  Bus Selector2/3 -> Degrees to Radians2/1  "<r>"
  Bus Selector/3 -> Mux1/3  "<w>"
  Bus Selector2/1 -> Degrees to Radians/1  "<p>"
  "     "/1(C_bv) -> Product/1  "C_bv"
  gravity [m/s^2]/1 -> Product/2  "g"
  Add1/1 -> Avoid_Low_Values/1(In)
  Degrees to Radians2/1 -> Mux/3  "r_rad_s"
  Add/1 -> Add1/1
  " "/1(skew(x)) -> Product2/1  "skew(omega_b)"
  [omega_b] -> " "/1(X)
  [InertiaTensor] -> Product2/2  "J_O_b"
  Degrees to Radians3/1 -> Bus Creator2/1  "phi_rad"
  Bus Selector1/2 -> Degrees to Radians4/1  "<theta>"
  Degrees to Radians1/1 -> Mux/2  "q_rad_s"
  Product/1 -> Product1/2  "g_b"
  Bus Selector/1 -> Mux1/1  "<u>"
  Degrees to Radians4/1 -> Bus Creator2/2  "theta_rad"
  Product3/1 -> Add/2
  [X] -> Bus Selector2/1, Bus Selector1/1, Bus Selector/1
  Product2/1 -> Add/1
  Bus Selector/2 -> Mux1/2  "<v>"
  Mux1/1 -> [V_b]  "V_b"
  Transpose/1 -> Product3/3  "V_b.'"
  Bus Selector2/2 -> Degrees to Radians1/1  "<q>"
  Mux/1 -> [omega_b]  "omega_b"
  [omega_b] -> Product2/3
  [omega_b] -> " 1"/1(X)
  "  "/1(skew(x)) -> Product4/2
  Center of Mass to Origin [m]/1 -> "  "/1(X)
  [Mass_kg] -> Product4/1
  Product4/1 -> [m_skew_rCb]
  [m_skew_rCb] -> Product1/1  "m*skew(rC_b)"
  X/1 -> [X]
  Bus Creator2/1 -> [att_rad]  "attitude_angles"
  [V_b] -> Transpose/1
  Moments_Nm/1 -> [M]
  [M] -> Add1/3
  " 1"/1(skew(x)) -> Product3/2  "skew(omega_b)"
  Avoid_Low_Values/1(Out) -> M_b/1

== system GenTil_Lib/GenTil/GenTil_Dynamics/Equations_of_Motion_6DoF/Dynamics/Rotation Matrix ==
  attitude_angles_rad : Inport
  Product1 : Product  Inputs=3  Multiplication=Matrix(*)
  Subsystem : Subsystem
  C_bv : Outport  PortDimensions=[3,3]
  C_phi : Outport  Port=2  PortDimensions=[3,3]
  wires:
  Subsystem/3(C_psi) -> Product1/3
  attitude_angles_rad/1 -> Subsystem/1(attitude_angles_rad)
  Product1/1 -> C_bv/1
  Subsystem/1(C_phi) -> Product1/1, C_phi/1
  Subsystem/2(C_theta) -> Product1/2

== system GenTil_Lib/GenTil/GenTil_Dynamics/Equations_of_Motion_6DoF/Dynamics/Translational and Rotational Kinematics ==
  note: 1.4-5
  X : Inport
  C_bv : Inport  Port=2
  C_phi : Inport  Port=3
  Bus Selector : BusSelector  OutputSignals=p,q,r
  Bus Selector2 : BusSelector  OutputSignals=u,v,w
  Constant : Constant
  Constant1 : Constant  Value=2
  Constant2 : Constant  Value=3
  Degrees to Radians : simulink_extras/Transformations/Degrees to Radians
  Degrees to Radians1 : simulink_extras/Transformations/Degrees to Radians
  Degrees to Radians2 : simulink_extras/Transformations/Degrees to Radians
  IdentityMatrix : IdentityMatrix  OutputDimensions=3
  Matrix Concatenate1 : Concatenate  NumInputs=3  Mode=Multidimensional array  ConcatenateDimension=2
  Matrix Concatenate2 : Concatenate  NumInputs=3  Mode=Multidimensional array
  Matrix Concatenate3 : Concatenate  NumInputs=3  Mode=Multidimensional array
  Matrix Divide : Product  Inputs=*/  Multiplication=Matrix(*)
  Matrix Multiply : Product  Multiplication=Matrix(*)
  Matrix Multiply1 : Product  Multiplication=Matrix(*)
  Radians to Degrees : simulink_extras/Transformations/Radians to Degrees
  Selector : Selector  NumberOfDimensions=2  InputPortWidth=3  IndexOptions=Select all,Index vector (port)  Indices=[2 3],1  OutputSizes=3,1
  Selector1 : Selector  NumberOfDimensions=2  InputPortWidth=3  IndexOptions=Select all,Index vector (port)  Indices=[2 3],1  OutputSizes=3,1
  Selector2 : Selector  NumberOfDimensions=2  InputPortWidth=3  IndexOptions=Select all,Index vector (port)  Indices=[2 3],1  OutputSizes=3,1
  Transpose : Math  Operator=transpose
  Phi_dot : Outport
  dReodt : Outport  Port=2
  wires:
  Matrix Concatenate3/1 -> Matrix Multiply1/2  "V_b"
  Matrix Multiply1/1 -> dReodt/1
  Matrix Divide/1 -> Matrix Multiply/1  "HPhi_inv"
  Selector2/1 -> Matrix Concatenate1/3
  C_phi/1 -> Selector/1, Selector1/1
  Bus Selector/3 -> Degrees to Radians2/1  "<r>"
  Selector1/1 -> Matrix Concatenate1/2
  Constant2/1 -> Selector2/2
  Constant1/1 -> Selector1/2
  Bus Selector2/1 -> Matrix Concatenate3/1  "<u>"
  X/1 -> Bus Selector/1, Bus Selector2/1
  Transpose/1 -> Matrix Multiply1/1  "C_bv.'"
  Radians to Degrees/1 -> Phi_dot/1  "Phi_dot"
  IdentityMatrix/1 -> Matrix Divide/1
  C_bv/1 -> Selector2/1, Transpose/1
  Bus Selector/2 -> Degrees to Radians1/1  "<q>"
  Constant/1 -> Selector/2
  Matrix Multiply/1 -> Radians to Degrees/1  "Phi_dot_rad"
  Matrix Concatenate2/1 -> Matrix Multiply/2  "omega_b"
  Matrix Concatenate1/1 -> Matrix Divide/2
  Bus Selector2/3 -> Matrix Concatenate3/3  "<w>"
  Degrees to Radians2/1 -> Matrix Concatenate2/3  "r_rad_s"
  Selector/1 -> Matrix Concatenate1/1
  Degrees to Radians1/1 -> Matrix Concatenate2/2  "q_rad_s"
  Bus Selector2/2 -> Matrix Concatenate3/2  "<v>"
  Degrees to Radians/1 -> Matrix Concatenate2/1  "p_rad_s"
  Bus Selector/1 -> Degrees to Radians/1  "<p>"

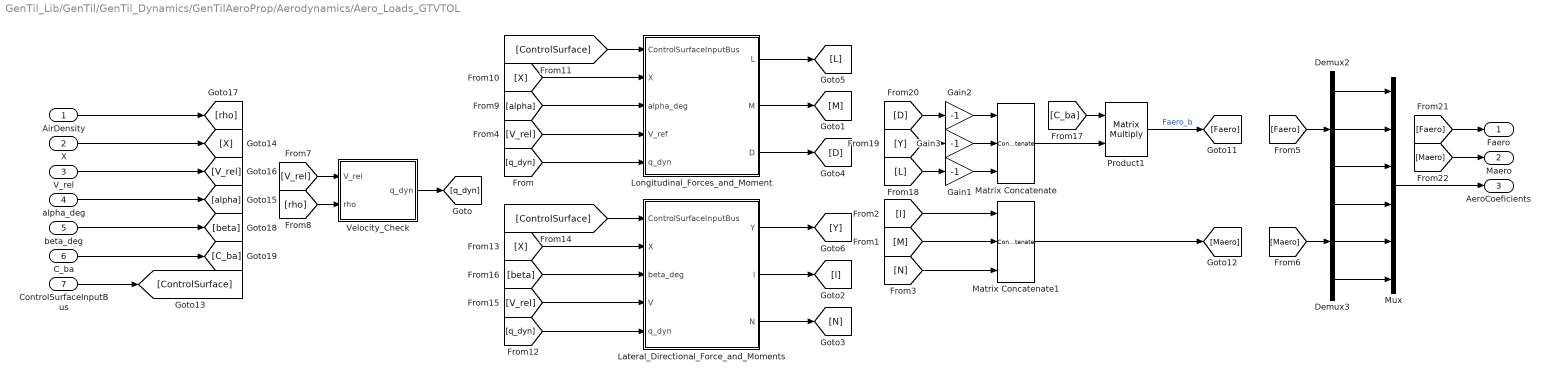
== system GenTil_Lib/GenTil/GenTil_Dynamics/GenTilAeroProp/Aerodynamics/Aero_Loads_GTVTOL ==
  AirDensity : Inport
  X : Inport  Port=2  OutDataTypeStr=Bus: States
  V_rel : Inport  Port=3
  alpha_deg : Inport  Port=4
  beta_deg : Inport  Port=5
  C_ba : Inport  Port=6
  ControlSurfaceInputBus : Inport  Port=7  OutDataTypeStr=Bus: Actuators
  Demux2 : Demux  Outputs=3
  Demux3 : Demux  Outputs=3
  Gain1 : Gain  Gain=-1
  Gain2 : Gain  Gain=-1
  Gain3 : Gain  Gain=-1
  Lateral_Directional_Force_and_Moments : Subsystem
  Longitudinal_Forces_and_Moment : Subsystem
  Matrix Concatenate : Concatenate  NumInputs=3  Mode=Multidimensional array
  Matrix Concatenate1 : Concatenate  NumInputs=3  Mode=Multidimensional array
  Mux : Mux  Inputs=6
  Product1 : Product  Multiplication=Matrix(*)
  Velocity_Check : Subsystem
  Faero : Outport
  Maero : Outport  Port=2
  AeroCoeficients : Outport  Port=3
  wires:
  [l] -> Matrix Concatenate1/1
  Matrix Concatenate/1 -> Product1/2
  Gain2/1 -> Matrix Concatenate/1
  Gain1/1 -> Matrix Concatenate/3
  [N] -> Matrix Concatenate1/3
  Matrix Concatenate1/1 -> [Maero]
  Gain3/1 -> Matrix Concatenate/2
  [M] -> Matrix Concatenate1/2
  Longitudinal_Forces_and_Moment/2(M) -> [M]
  beta_deg/1 -> [beta]
  C_ba/1 -> [C_ba]
  Demux2/2 -> Mux/2
  Mux/1 -> AeroCoeficients/1
  Demux2/3 -> Mux/3
  Demux3/1 -> Mux/4
  Demux2/1 -> Mux/1
  Demux3/3 -> Mux/6
  Demux3/2 -> Mux/5
  Product1/1 -> [Faero]  "Faero_b"
  [Faero] -> Demux2/1
  [Maero] -> Demux3/1
  ControlSurfaceInputBus/1 -> [ControlSurface]
  X/1 -> [X]
  alpha_deg/1 -> [alpha]
  V_rel/1 -> [V_rel]
  AirDensity/1 -> [rho]
  Longitudinal_Forces_and_Moment/3(D) -> [D]
  Longitudinal_Forces_and_Moment/1(L) -> [L]
  [ControlSurface] -> Longitudinal_Forces_and_Moment/1(ControlSurfaceInputBus)
  [X] -> Longitudinal_Forces_and_Moment/2(X)
  [alpha] -> Longitudinal_Forces_and_Moment/3(alpha_deg)
  [V_rel] -> Longitudinal_Forces_and_Moment/4(V_ref)
  [q_dyn] -> Longitudinal_Forces_and_Moment/5(q_dyn)
  [ControlSurface] -> Lateral_Directional_Force_and_Moments/1(ControlSurfaceInputBus)
  [X] -> Lateral_Directional_Force_and_Moments/2(X)
  [beta] -> Lateral_Directional_Force_and_Moments/3(beta_deg)
  [V_rel] -> Lateral_Directional_Force_and_Moments/4(V)
  [q_dyn] -> Lateral_Directional_Force_and_Moments/5(q_dyn)
  Lateral_Directional_Force_and_Moments/2(l) -> [l]
  Lateral_Directional_Force_and_Moments/3(N) -> [N]
  Lateral_Directional_Force_and_Moments/1(Y) -> [Y]
  [C_ba] -> Product1/1
  [L] -> Gain1/1
  [Y] -> Gain3/1
  [D] -> Gain2/1
  [Faero] -> Faero/1
  [Maero] -> Maero/1
  [V_rel] -> Velocity_Check/1(V_rel)
  [rho] -> Velocity_Check/2(rho)
  Velocity_Check/1(q_dyn) -> [q_dyn]

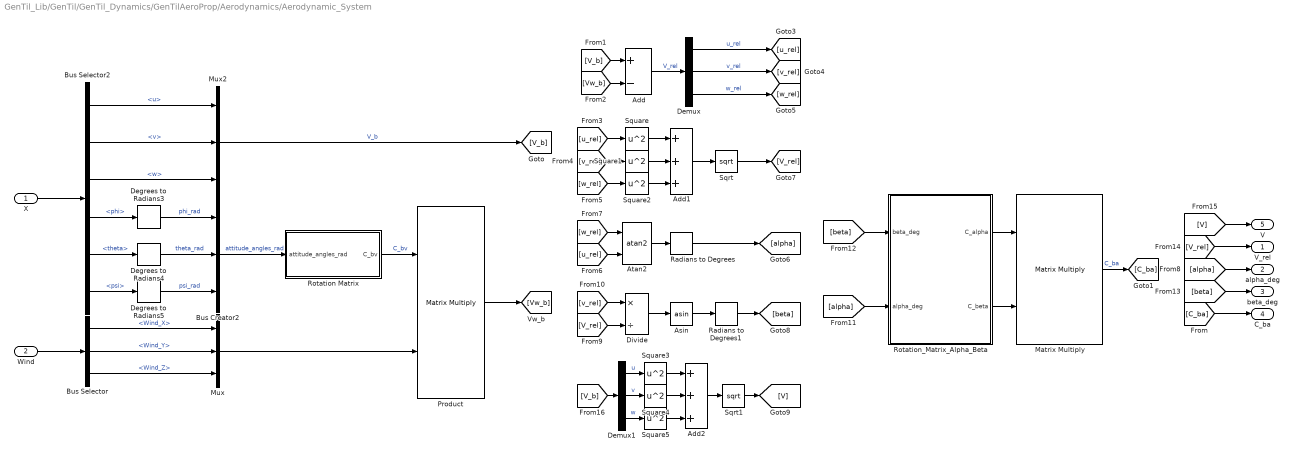
== system GenTil_Lib/GenTil/GenTil_Dynamics/GenTilAeroProp/Aerodynamics/Aerodynamic_System ==
  X : Inport  OutDataTypeStr=Bus: States
  Wind : Inport  Port=2
  Add : Sum  Inputs=+-
  Add1 : Sum  Inputs=3
  Add2 : Sum  Inputs=3
  Asin : Trigonometry  Operator=asin
  Atan2 : Trigonometry  Operator=atan2
  Bus Creator2 : BusCreator  Inputs=3
  Bus Selector : BusSelector  OutputSignals=Wind_X,Wind_Y,Wind_Z
  Bus Selector2 : BusSelector  OutputSignals=u,v,w,phi,theta,psi
  Degrees to Radians3 : simulink_extras/Transformations/Degrees to Radians
  Degrees to Radians4 : simulink_extras/Transformations/Degrees to Radians
  Degrees to Radians5 : simulink_extras/Transformations/Degrees to Radians
  Demux : Demux  Outputs=3
  Demux1 : Demux  Outputs=3
  Divide : Product  Inputs=*/
  Matrix Multiply : Product  Multiplication=Matrix(*)
  Mux : Mux  Inputs=3
  Mux2 : Mux  Inputs=3
  Product : Product  Multiplication=Matrix(*)
  Radians to Degrees : simulink_extras/Transformations/Radians to Degrees
  Radians to Degrees1 : simulink_extras/Transformations/Radians to Degrees
  Rotation Matrix : Subsystem
  Rotation_Matrix_Alpha_Beta : Subsystem
  Sqrt : Sqrt
  Sqrt1 : Sqrt
  Square{,1..5} (6 alike) : Math  Operator=square
  V_rel : Outport
  alpha_deg : Outport  Port=2
  beta_deg : Outport  Port=3
  C_ba : Outport  Port=4
  V : Outport  Port=5
  wires:
  Mux2/1 -> [V_b]  "V_b"
  Product/1 -> [Vw_b]
  Mux/1 -> Product/2
  Bus Selector/3 -> Mux/3  "<Wind_Z>"
  Bus Selector/2 -> Mux/2  "<Wind_Y>"
  Bus Selector/1 -> Mux/1  "<Wind_X>"
  Bus Selector2/5 -> Degrees to Radians4/1  "<theta>"
  Degrees to Radians3/1 -> Bus Creator2/1  "phi_rad"
  Degrees to Radians5/1 -> Bus Creator2/3  "psi_rad"
  Degrees to Radians4/1 -> Bus Creator2/2  "theta_rad"
  Bus Selector2/4 -> Degrees to Radians3/1  "<phi>"
  Bus Selector2/6 -> Degrees to Radians5/1  "<psi>"
  Bus Creator2/1 -> Rotation Matrix/1(attitude_angles_rad)  "attitude_angles_rad"
  Rotation Matrix/1(C_bv) -> Product/1  "C_bv"
  Wind/1 -> Bus Selector/1
  Rotation_Matrix_Alpha_Beta/2(C_beta) -> Matrix Multiply/2
  Matrix Multiply/1 -> [C_ba]  "C_ba"
  Rotation_Matrix_Alpha_Beta/1(C_alpha) -> Matrix Multiply/1
  X/1 -> Bus Selector2/1
  Bus Selector2/3 -> Mux2/3  "<w>"
  Bus Selector2/2 -> Mux2/2  "<v>"
  Bus Selector2/1 -> Mux2/1  "<u>"
  [C_ba] -> C_ba/1
  [V_b] -> Add/1
  [Vw_b] -> Add/2
  Demux/3 -> [w_rel]  "w_rel"
  Demux/2 -> [v_rel]  "v_rel"
  Demux/1 -> [u_rel]  "u_rel"
  Add/1 -> Demux/1  "V_rel"
  Atan2/1 -> Radians to Degrees/1
  [w_rel] -> Atan2/1
  [u_rel] -> Atan2/2
  Radians to Degrees/1 -> [alpha]
  [alpha] -> alpha_deg/1
  [w_rel] -> Square2/1
  Square1/1 -> Add1/2
  Square2/1 -> Add1/3
  [v_rel] -> Square1/1
  Square/1 -> Add1/1
  Sqrt/1 -> [V_rel]
  [u_rel] -> Square/1
  Add1/1 -> Sqrt/1
  Asin/1 -> Radians to Degrees1/1
  [v_rel] -> Divide/1
  [V_rel] -> Divide/2
  Divide/1 -> Asin/1
  Radians to Degrees1/1 -> [beta]
  [alpha] -> Rotation_Matrix_Alpha_Beta/2(alpha_deg)
  [beta] -> Rotation_Matrix_Alpha_Beta/1(beta_deg)
  [beta] -> beta_deg/1
  [V_rel] -> V_rel/1
  [V] -> V/1
  [V_b] -> Demux1/1
  Add2/1 -> Sqrt1/1
  Sqrt1/1 -> [V]
  Square3/1 -> Add2/1
  Square5/1 -> Add2/3
  Square4/1 -> Add2/2
  Demux1/1 -> Square3/1  "u"
  Demux1/2 -> Square4/1  "v"
  Demux1/3 -> Square5/1  "w"

== system GenTil_Lib/GenTil/GenTil_Dynamics/Equations_of_Motion_6DoF/Dynamics/Forces/Avoid_Low_Values ==
  In : Inport
  Abs : Abs  SaturateOnIntegerOverflow=off
  Compare To Constant : simulink/Logic and Bit Operations/Compare To Constant  relop=<  const=1e-4  OutDataTypeStr=boolean
  Constant : Constant  Value=0  SampleTime=-1
  Data Type Conversion : DataTypeConversion  OutDataTypeStr=double  SaturateOnIntegerOverflow=off  RndMeth=Floor
  Switch : Switch  Criteria=u2 > Threshold  Threshold=0.05  SaturateOnIntegerOverflow=off  InputSameDT=off
  Out : Outport
  wires:
  Constant/1 -> Switch/1
  Abs/1 -> Compare To Constant/1
  Compare To Constant/1 -> Data Type Conversion/1
  In/1 -> Switch/3, Abs/1
  Data Type Conversion/1 -> Switch/2
  Switch/1 -> Out/1

== system GenTil_Lib/GenTil/GenTil_Dynamics/Equations_of_Motion_6DoF/Dynamics/Forces/Rotation Matrix ==
  attitude_angles_rad : Inport
  Product1 : Product  Inputs=3  Multiplication=Matrix(*)
  Subsystem : Subsystem
  C_bv : Outport  PortDimensions=[3,3]
  wires:
  attitude_angles_rad/1 -> Subsystem/1(attitude_angles_rad)
  Product1/1 -> C_bv/1
  Subsystem/3(C_psi) -> Product1/3
  Subsystem/1(C_phi) -> Product1/1
  Subsystem/2(C_theta) -> Product1/2

== system GenTil_Lib/GenTil/GenTil_Dynamics/Equations_of_Motion_6DoF/Dynamics/Forces/Skew ==
  note: In mathematics, a skew symmetric matrix is defined as the square matrix that is equal to the negative of its transpose matrix.
      | For any square matrix, A, the transpose matrix is given as A T . A skew-symmetric or antisymmetric matrix A can therefore be represented as, A = -A T .
  X : Inport
  Constant : Constant  Value=0
  Constant1 : Constant  Value=0
  Constant2 : Constant  Value=0
  Demux : Demux  Outputs=3
  From : From
  From1 : From
  Gain3 : Gain  Gain=-1
  Gain4 : Gain  Gain=-1
  Gain5 : Gain  Gain=-1
  Goto : Goto
  Matrix Concatenate3 : Concatenate  NumInputs=3  Mode=Multidimensional array  ConcatenateDimension=2
  Matrix Concatenate4 : Concatenate  NumInputs=3  Mode=Multidimensional array  ConcatenateDimension=2
  Matrix Concatenate5 : Concatenate  NumInputs=3  Mode=Multidimensional array  ConcatenateDimension=2
  Matrix Concatenate6 : Concatenate  NumInputs=3  Mode=Multidimensional array
  skew(x) : Outport
  wires:
  Constant2/1 -> Matrix Concatenate5/3
  Constant1/1 -> Matrix Concatenate4/2
  Constant/1 -> Matrix Concatenate3/1
  Demux/1 -> Goto/1
  Demux/2 -> [B]
  X/1 -> Demux/1
  [B] -> Gain4/1
  From1/1 -> Matrix Concatenate5/2
  Matrix Concatenate3/1 -> Matrix Concatenate6/1
  Demux/3 -> [C]
  [B] -> Matrix Concatenate3/3
  Matrix Concatenate5/1 -> Matrix Concatenate6/3
  Matrix Concatenate6/1 -> skew(x)/1  "skew(x)"
  Gain4/1 -> Matrix Concatenate5/1
  [C] -> Gain5/1
  [C] -> Matrix Concatenate4/1
  Gain3/1 -> Matrix Concatenate4/3
  From/1 -> Gain3/1
  Matrix Concatenate4/1 -> Matrix Concatenate6/2
  Gain5/1 -> Matrix Concatenate3/2

== system GenTil_Lib/GenTil/GenTil_Dynamics/Equations_of_Motion_6DoF/Dynamics/Forces/Skew1 ==
  note: In mathematics, a skew symmetric matrix is defined as the square matrix that is equal to the negative of its transpose matrix.
      | For any square matrix, A, the transpose matrix is given as A T . A skew-symmetric or antisymmetric matrix A can therefore be represented as, A = -A T .
  X : Inport
  Constant : Constant  Value=0
  Constant1 : Constant  Value=0
  Constant2 : Constant  Value=0
  Demux : Demux  Outputs=3
  From : From
  From1 : From
  Gain3 : Gain  Gain=-1
  Gain4 : Gain  Gain=-1
  Gain5 : Gain  Gain=-1
  Goto : Goto
  Matrix Concatenate3 : Concatenate  NumInputs=3  Mode=Multidimensional array  ConcatenateDimension=2
  Matrix Concatenate4 : Concatenate  NumInputs=3  Mode=Multidimensional array  ConcatenateDimension=2
  Matrix Concatenate5 : Concatenate  NumInputs=3  Mode=Multidimensional array  ConcatenateDimension=2
  Matrix Concatenate6 : Concatenate  NumInputs=3  Mode=Multidimensional array
  skew(x) : Outport
  wires:
  Constant2/1 -> Matrix Concatenate5/3
  Constant1/1 -> Matrix Concatenate4/2
  Constant/1 -> Matrix Concatenate3/1
  Demux/1 -> Goto/1
  Demux/2 -> [B]
  X/1 -> Demux/1
  [B] -> Gain4/1
  From1/1 -> Matrix Concatenate5/2
  Matrix Concatenate3/1 -> Matrix Concatenate6/1
  Demux/3 -> [C]
  [B] -> Matrix Concatenate3/3
  Matrix Concatenate5/1 -> Matrix Concatenate6/3
  Matrix Concatenate6/1 -> skew(x)/1  "skew(x)"
  Gain4/1 -> Matrix Concatenate5/1
  [C] -> Gain5/1
  [C] -> Matrix Concatenate4/1
  Gain3/1 -> Matrix Concatenate4/3
  From/1 -> Gain3/1
  Matrix Concatenate4/1 -> Matrix Concatenate6/2
  Gain5/1 -> Matrix Concatenate3/2

== system GenTil_Lib/GenTil/GenTil_Dynamics/Equations_of_Motion_6DoF/Dynamics/Generalized Mass Matrix/Skew ==
  note: In mathematics, a skew symmetric matrix is defined as the square matrix that is equal to the negative of its transpose matrix.
      | For any square matrix, A, the transpose matrix is given as A T . A skew-symmetric or antisymmetric matrix A can therefore be represented as, A = -A T .
  X : Inport
  Constant : Constant  Value=0
  Constant1 : Constant  Value=0
  Constant2 : Constant  Value=0
  Demux : Demux  Outputs=3
  From : From
  From1 : From
  Gain3 : Gain  Gain=-1
  Gain4 : Gain  Gain=-1
  Gain5 : Gain  Gain=-1
  Goto : Goto
  Matrix Concatenate3 : Concatenate  NumInputs=3  Mode=Multidimensional array  ConcatenateDimension=2
  Matrix Concatenate4 : Concatenate  NumInputs=3  Mode=Multidimensional array  ConcatenateDimension=2
  Matrix Concatenate5 : Concatenate  NumInputs=3  Mode=Multidimensional array  ConcatenateDimension=2
  Matrix Concatenate6 : Concatenate  NumInputs=3  Mode=Multidimensional array
  skew(x) : Outport
  wires:
  Constant2/1 -> Matrix Concatenate5/3
  Constant1/1 -> Matrix Concatenate4/2
  Constant/1 -> Matrix Concatenate3/1
  Demux/1 -> Goto/1
  Demux/2 -> [B]
  X/1 -> Demux/1
  [B] -> Gain4/1
  From1/1 -> Matrix Concatenate5/2
  Matrix Concatenate3/1 -> Matrix Concatenate6/1
  Demux/3 -> [C]
  [B] -> Matrix Concatenate3/3
  Matrix Concatenate5/1 -> Matrix Concatenate6/3
  Matrix Concatenate6/1 -> skew(x)/1  "skew(x)"
  Gain4/1 -> Matrix Concatenate5/1
  [C] -> Gain5/1
  [C] -> Matrix Concatenate4/1
  Gain3/1 -> Matrix Concatenate4/3
  From/1 -> Gain3/1
  Matrix Concatenate4/1 -> Matrix Concatenate6/2
  Gain5/1 -> Matrix Concatenate3/2
